simulink library "optimizeThrLenghtAndElevation_ul"  (R2020a)
settings: Solver=VariableStepAuto  StartTime=0.0  StopTime=10.0  RelTol=1e-3
values from neighbouring files (symbols this model uses):
  hiLvlCtrl = block.DialogPrm(2).Data    [optimizeAltitude_Lvl2SFun.m]    (also in optimizeThrLenghtAndElevation_Lvl2sFun.m; optimizeTrajectory_Lvl2SFun.m)
  midLvlKfgp = GP.KalmanFilteredGaussianProcess(hiLvlCtrl.spatialCovFn,     hiLvlCtrl.temporalCovFn,hiLvlCtrl.meanFn,hiLvlCtrl.xMeasure,     hiLvlCtrl.midLvlCtrl.dt)    [midLvlCtrlKfgp_init.m]    (also in optimizeThrLenghtAndElevation_Lvl2sFun.m = block.DialogPrm(1).Data)
libraries: dspsigops x3
settings Model: Creator=Ayaz  LastModifiedBy=Ayaz

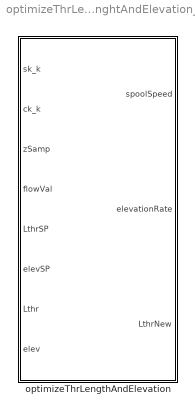
== system optimizeThrLenghtAndElevation_ul ==
  optimizeThrLengthAndElevation : Subsystem  mask{hiLvlCtrl=hiLvlCtrl}
      mask prompts: hiLvlCtrl "High level controller object"
      mask TypeOptions hiLvlCtrl: optimizeThrLengthAndElevationTraj/hiLvlCtrl

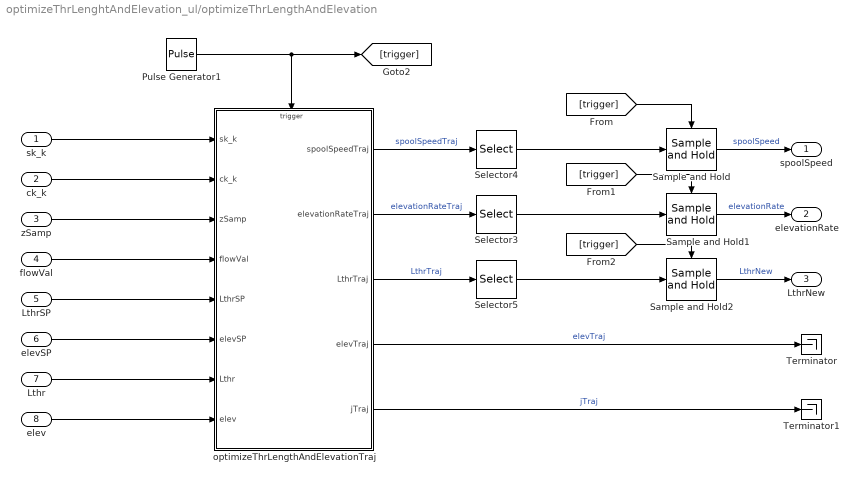
== system optimizeThrLenghtAndElevation_ul/optimizeThrLengthAndElevation ==
  sk_k : Inport
  ck_k : Inport  Port=2
  zSamp : Inport  Port=3
  flowVal : Inport  Port=4
  LthrSP : Inport  Port=5
  elevSP : Inport  Port=6
  Lthr : Inport  Port=7
  elev : Inport  Port=8
  Pulse Generator1 : DiscretePulseGenerator  PulseType=Time based  Period=hiLvlCtrl.midLvlCtrl.dt*60  PhaseDelay=hiLvlCtrl.mpckfgpTimeStep*60
  Sample and Hold : dspsigops/Sample and Hold  trig=Rising edge  initCond=0  latchinput=off
  Sample and Hold1 : dspsigops/Sample and Hold  trig=Rising edge  initCond=0  latchinput=off
  Sample and Hold2 : dspsigops/Sample and Hold  trig=Rising edge  initCond=hiLvlCtrl.initVals(3)  latchinput=off
  Selector3 : Selector  InputPortWidth=hiLvlCtrl.midLvlCtrl.predHorz  IndexOptions=Index vector (dialog)  Indices=1  OutputSizes=1
  Selector4 : Selector  InputPortWidth=hiLvlCtrl.midLvlCtrl.predHorz  IndexOptions=Index vector (dialog)  Indices=1  OutputSizes=1
  Selector5 : Selector  InputPortWidth=hiLvlCtrl.midLvlCtrl.predHorz  IndexOptions=Index vector (dialog)  Indices=1  OutputSizes=1
  Terminator : Terminator
  Terminator1 : Terminator
  optimizeThrLengthAndElevationTraj : Subsystem  mask{hiLvlCtrl=hiLvlCtrl}
      mask prompts: hiLvlCtrl "High level controller object"
      mask init:
      | midLvlCtrlKfgp_init
  spoolSpeed : Outport
  elevationRate : Outport  Port=2
  LthrNew : Outport  Port=3
  wires:
  optimizeThrLengthAndElevationTraj/2(elevationRateTraj) -> Selector3/1  "elevationRateTraj"
  optimizeThrLengthAndElevationTraj/1(spoolSpeedTraj) -> Selector4/1  "spoolSpeedTraj"
  optimizeThrLengthAndElevationTraj/4(elevTraj) -> Terminator/1  "elevTraj"
  optimizeThrLengthAndElevationTraj/5(jTraj) -> Terminator1/1  "jTraj"
  optimizeThrLengthAndElevationTraj/3(LthrTraj) -> Selector5/1  "LthrTraj"
  Lthr/1 -> optimizeThrLengthAndElevationTraj/7(Lthr)
  LthrSP/1 -> optimizeThrLengthAndElevationTraj/5(LthrSP)
  elev/1 -> optimizeThrLengthAndElevationTraj/8(elev)
  flowVal/1 -> optimizeThrLengthAndElevationTraj/4(flowVal)
  elevSP/1 -> optimizeThrLengthAndElevationTraj/6(elevSP)
  ck_k/1 -> optimizeThrLengthAndElevationTraj/2(ck_k)
  zSamp/1 -> optimizeThrLengthAndElevationTraj/3(zSamp)
  sk_k/1 -> optimizeThrLengthAndElevationTraj/1(sk_k)
  Pulse Generator1/1 -> [trigger], optimizeThrLengthAndElevationTraj/Trigger
  Sample and Hold/1 -> spoolSpeed/1  "spoolSpeed"
  [trigger] -> Sample and Hold/Trigger
  Sample and Hold1/1 -> elevationRate/1  "elevationRate"
  [trigger] -> Sample and Hold1/Trigger
  Sample and Hold2/1 -> LthrNew/1  "LthrNew"
  [trigger] -> Sample and Hold2/Trigger
  Selector4/1 -> Sample and Hold/1
  Selector3/1 -> Sample and Hold1/1
  Selector5/1 -> Sample and Hold2/1

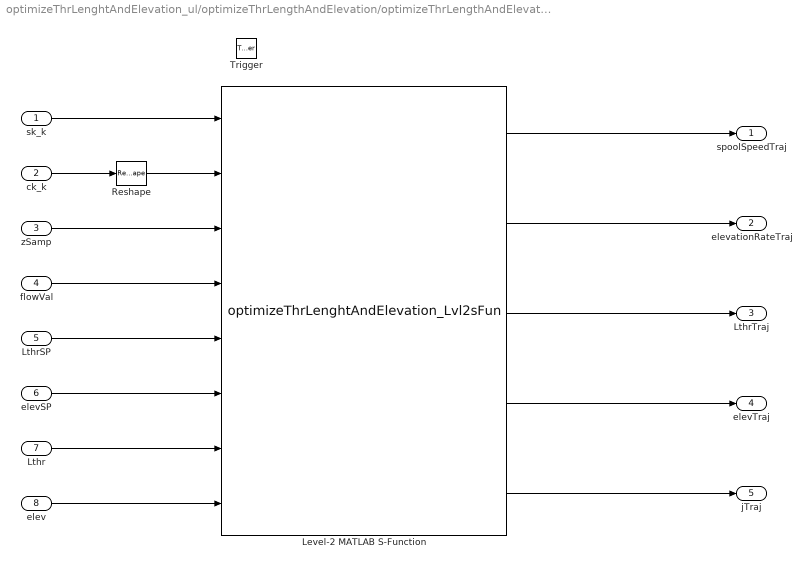
== system optimizeThrLenghtAndElevation_ul/optimizeThrLengthAndElevation/optimizeThrLengthAndElevationTraj ==
  sk_k : Inport
  ck_k : Inport  Port=2
  zSamp : Inport  Port=3
  flowVal : Inport  Port=4
  LthrSP : Inport  Port=5
  elevSP : Inport  Port=6
  Lthr : Inport  Port=7
  elev : Inport  Port=8
  Trigger : TriggerPort  VariantControl=Variant
  Level-2 MATLAB S-Function : M-S-Function  FunctionName=optimizeThrLenghtAndElevation_Lvl2sFun  Parameters=midLvlKfgp,hiLvlCtrl
  Reshape : Reshape  OutputDimensionality=Column vector (2-D)
  spoolSpeedTraj : Outport
  elevationRateTraj : Outport  Port=2
  LthrTraj : Outport  Port=3
  elevTraj : Outport  Port=4
  jTraj : Outport  Port=5
  wires:
  flowVal/1 -> Level-2 MATLAB S-Function/4
  zSamp/1 -> Level-2 MATLAB S-Function/3
  ck_k/1 -> Reshape/1
  sk_k/1 -> Level-2 MATLAB S-Function/1
  Reshape/1 -> Level-2 MATLAB S-Function/2
  LthrSP/1 -> Level-2 MATLAB S-Function/5
  elevSP/1 -> Level-2 MATLAB S-Function/6
  Lthr/1 -> Level-2 MATLAB S-Function/7
  elev/1 -> Level-2 MATLAB S-Function/8
  Level-2 MATLAB S-Function/1 -> spoolSpeedTraj/1
  Level-2 MATLAB S-Function/5 -> jTraj/1
  Level-2 MATLAB S-Function/2 -> elevationRateTraj/1
  Level-2 MATLAB S-Function/3 -> LthrTraj/1
  Level-2 MATLAB S-Function/4 -> elevTraj/1
